simulink model "DSB_SC_AM_system_with_awgn"  (R2021a)
settings: Solver=VariableStepAuto  StartTime=0.0  StopTime=10  RelTol=1e-3
libraries: dsparch4 x1, simulink x1
settings Model: Creator=Fatiha  LastModifiedBy=Fatiha

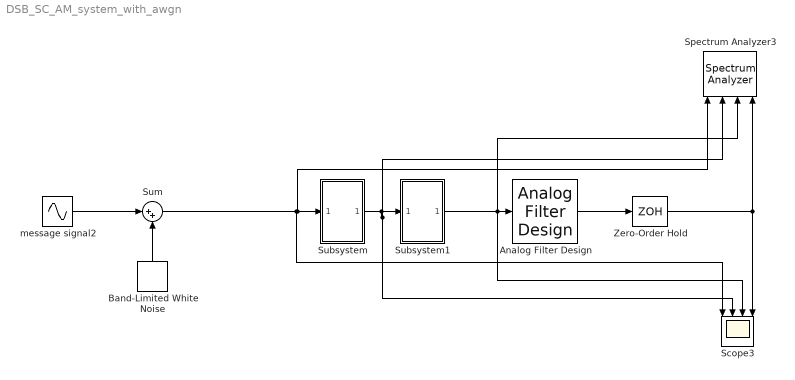
== system DSB_SC_AM_system_with_awgn ==
  Analog Filter Design : dsparch4/Analog Filter Design  method=Butterworth  filttype=Lowpass  N=8  Wlo=2*pi*0.5e3  Whi=80  Rp=2  Rs=40
  Band-Limited White Noise : simulink/Sources/Band-Limited White Noise  Cov=[1e-8]  Ts=1/50000  seed=[23341]
  Scope3 : Scope  NumInputPorts=4
  Spectrum Analyzer3 : SpectrumAnalyzer  NumInputPorts=4
  Subsystem : Subsystem
  Subsystem1 : Subsystem
  Sum : Sum  Inputs=|++
  Zero-Order Hold : ZeroOrderHold  SampleTime=-1
  message signal2 : Sin  Bias=5  Frequency=2*pi*50  Phase=pi/2  SampleTime=1/50000
  wires:
  Sum/1 -> Spectrum Analyzer3/1, Subsystem/1(In1), Scope3/1
  Subsystem/1(Out1) -> Spectrum Analyzer3/2, Scope3/2, Subsystem1/1(In1)
  Subsystem1/1(Out1) -> Scope3/3, Spectrum Analyzer3/3, Analog Filter Design/1
  Analog Filter Design/1 -> Zero-Order Hold/1
  Zero-Order Hold/1 -> Scope3/4, Spectrum Analyzer3/4
  message signal2/1 -> Sum/1
  Band-Limited White Noise/1 -> Sum/2

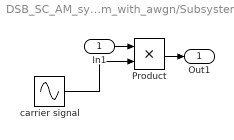
== system DSB_SC_AM_system_with_awgn/Subsystem ==
  In1 : Inport
  Product : Product
  carrier signal : Sin  Frequency=2*pi*500  Phase=pi/2  SampleTime=1/50000
  Out1 : Outport
  wires:
  carrier signal/1 -> Product/2
  Product/1 -> Out1/1
  In1/1 -> Product/1

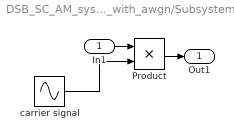
== system DSB_SC_AM_system_with_awgn/Subsystem1 ==
  In1 : Inport
  Product : Product
  carrier signal : Sin  Frequency=2*pi*500  Phase=pi/2  SampleTime=1/50000
  Out1 : Outport
  wires:
  carrier signal/1 -> Product/2
  Product/1 -> Out1/1
  In1/1 -> Product/1
